simulink model "fskmod"  (R2014b)
settings: Solver=ode45  StartTime=0.0  StopTime=10.0  RelTol=1e-3
InitFcn:
  | samp_per_frame = 32;
  | fs = 1000000;
  | samp_per_sym = 16;
  | BT = 0.5;
  | mod_index = 0.33;
libraries: rfmathmodels1 x1, commrandsrc2 x1, commobslib x1, commdigbbndfm2 x1
settings Model: Creator=Ben  LastModifiedBy=Ben

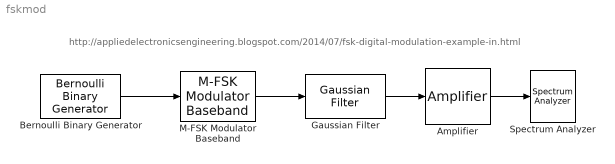
== system fskmod ==
  note: http://appliedelectronicsengineering.blogspot.com/2014/07/fsk-digital-modulation-example-in.html
  Amplifier : rfmathmodels1/Amplifier  model_select=Linear  linGaindB=-90  GindB=0  iip3=30  am2pm=10  PwrAMPMStart=10  PwrAMPMEnd=inf  amam=[2.1587 1.1517]  ampm=[4.0033 9.1040]  x=[8.1081 1.5413 6.5202 -0.0718]  y=[4.6645 2.0965 10.88 -0.003]  p=0.5  GoutdB=0  vsat=1  method_select=Noise factor  ntemp=290  nfigure=3.01  nfactor=2  seed=67987
  Bernoulli Binary Generator : commrandsrc2/Bernoulli Binary Generator  P=0.5  seed=11  Ts=1/fs  frameBased=on  sampPerFrame=samp_per_frame  orient=off  outDataType=double
  Gaussian Filter : commobslib/Gaussian Filter  N=samp_per_sym  BT=BT  D=1  sampMode=Frame-based  normMode=Sum of coefficients  filterGain=1  checkCoeff=off  variableName=gaussFilt  launchFVT=off  roundingMode=Floor  overflowMode=off  InputProcessing=Columns as channels (frame based)
  M-FSK Modulator Baseband : commdigbbndfm2/M-FSK Modulator Baseband  M=2  InType=Integer  Enc=Binary  freqSep=mod_index*fs  phaseType=Continuous  numSamp=16  RateOptions=Enforce single-rate processing  outDataType=double
  Spectrum Analyzer : SpectrumAnalyzer
  wires:
  Bernoulli Binary Generator/1 -> M-FSK Modulator Baseband/1
  M-FSK Modulator Baseband/1 -> Gaussian Filter/1
  Gaussian Filter/1 -> Amplifier/1
  Amplifier/1 -> Spectrum Analyzer/1
